simulink model "cosmic_ray_system"  (R2019a)
settings: Solver=VariableStepAuto  StartTime=0.0  StopTime=1000  RelTol=1e-3
libraries: xbsIndex_r4 x6191, casper_library_misc x163, xps_library x4, casper_library_delays x4
(part 15 of 40)

== system cosmic_ray_system/cosmic_ray/coincidence_trigger/trigger_coincidencer ==
  window_length : Inport
  data_bus_in : Inport  Port=2
  sync_in : Inport  Port=3
  adder_tree : Subsystem  AncestorBlock=casper_library_misc/adder_tree  mask(adder_tree){n_inputs=64, csp_latency=1, adder_imp=Fabric, first_stage_hdl=on, floating_point=off, dvalid_en=off, float_type=single, frac_width=0, exp_width=0}
      mask prompts: n_inputs "Number of Inputs"; csp_latency "Add Latency"; adder_imp "Adder implementation"; first_stage_hdl "Use behavioural HDL for first stage of adders"; floating_point "floating point"; float_type "float type"; frac_width "fraction length"; exp_width "exponent length"
      mask help:
      | Sums all inputs using a tree of adds and delays.
      |
      | Number of inputs: The number of inputs to the block to be summed
      | Add latency: The number of clock cycles to perform one addition (affects timing)..
      | Adder implementation: choice of fabric or DSP48E core, or behavioral HDL
      | Use behavioural HDL for first stage of adders: Causes the first stage of adders to be absorbed into DSP blocks if multipliers precede them (Virtex 5). Overrides Adder implementation
      mask init:
      | adder_tree_init(gcb, ...
      |     'n_inputs', n_inputs, ...
      |     'csp_latency', csp_latency, ...
      |     'adder_imp', adder_imp, ...
      |     'dvalid_en', dvalid_en, ...
      |     'floating_point', floating_point, ...
      |     'float_type', float_type, ...
      |     'exp_width', exp_width, ...
      |     'frac_width', frac_width, ...     
      |     'first_stage_hdl', first_stage_hdl);
      settings: AttributesFormatString=latency 6
      mask Help: eval('xlWeb(''http://casper.berkeley.edu/wiki/Adder_tree'')')
      mask TypeOptions adder_imp: Behavioral | Fabric | DSP48
      mask Callback floating_point:
      | onoff = get_param(gcb, 'floating_point');
      | if strcmp(onoff,'on')
      |     enable_fixpt = 'off'
      |     set_param_state(gcb, 'float_type', 'on')
      | 
      |     f_type = get_param(gcb, 'float_type')
      |     if strcmp(f_type,'custom')
      |         set_param_state(gcb, 'exp_width', 'on')
      |         set_param_state(gcb, 'frac_width', 'on')
      |     else
      |         set_param_state(gcb, 'exp_width', 'off')
      |         set_param_state(gcb, 'frac_width', 'off')
      |     end
      | 
      | 
      | else
      |     enable_fixpt = 'on'
      |     set_param_state(gcb, 'float_type', 'off')
      |     set_param_state(gcb, 'exp_width', 'off')
      |     set_param_state(gcb, 'frac_width', 'off')
      | end
      mask TypeOptions float_type: single | custom
      mask Callback float_type:
      | f_type = get_param(gcb, 'float_type')
      | if strcmp(f_type,'custom')
      |     set_param_state(gcb, 'exp_width', 'on')
      |     set_param_state(gcb, 'frac_width', 'on')
      | else
      |     set_param_state(gcb, 'exp_width', 'off')
      |     set_param_state(gcb, 'frac_width', 'off')
      | end
  bus_expand : Subsystem  AncestorBlock=casper_library_flow_control/bus_expand  mask(bus_expand){mode=divisions of equal size, outputNum=64, outputWidth=1, outputBinaryPt=0, outputArithmeticType=0, show_format=off, outputToWorkspace=off, variablePrefix=out, outputToModelAsWell=on}
      mask prompts: outputNum "Number of outputs:"; outputWidth "Output width:"; outputBinaryPt "Output binary point position:"; outputArithmeticType "Output arithmetic type (ufix=0, fix=1, bool=2):"; show_format "Print format string?"; outputToWorkspace "Output to workspace?"; variablePrefix "Variable name prefix:"; outputToModelAsWell "Output to model as well?"
      mask help:
      | Expands a 'bus' made using a bus_create or Xilinx
      | concat block.
      | The input will be divided into the specified number
      | of outputs with the specified arithmetic types.
      | Divisions are made from most significant bit.
      mask init: same as cosmic_ray_system/cosmic_ray/buffer_and_packetizer/bus_expand1
      settings: AttributesFormatString=64 outputs
      mask TypeOptions mode: divisions of equal size | divisions of arbitrary size
      mask Callback mode: bus_expand_callback();
      mask Callback outputWidth: bus_expand_callback();
      mask Callback outputToWorkspace: bus_expand_callback();
  custom_pulse_extend1 : Subsystem
  custom_pulse_extend10 : Subsystem
  custom_pulse_extend11 : Subsystem
  custom_pulse_extend12 : Subsystem
  custom_pulse_extend13 : Subsystem
  custom_pulse_extend14 : Subsystem
  custom_pulse_extend15 : Subsystem
  custom_pulse_extend16 : Subsystem
  custom_pulse_extend17 : Subsystem
  custom_pulse_extend18 : Subsystem
  custom_pulse_extend19 : Subsystem
  custom_pulse_extend2 : Subsystem
  custom_pulse_extend20 : Subsystem
  custom_pulse_extend21 : Subsystem
  custom_pulse_extend22 : Subsystem
  custom_pulse_extend23 : Subsystem
  custom_pulse_extend24 : Subsystem
  custom_pulse_extend25 : Subsystem
  custom_pulse_extend26 : Subsystem
  custom_pulse_extend27 : Subsystem
  custom_pulse_extend28 : Subsystem
  custom_pulse_extend29 : Subsystem
  custom_pulse_extend3 : Subsystem
  custom_pulse_extend30 : Subsystem
  custom_pulse_extend31 : Subsystem
  custom_pulse_extend32 : Subsystem
  custom_pulse_extend33 : Subsystem
  custom_pulse_extend34 : Subsystem
  custom_pulse_extend35 : Subsystem
  custom_pulse_extend36 : Subsystem
  custom_pulse_extend37 : Subsystem
  custom_pulse_extend38 : Subsystem
  custom_pulse_extend39 : Subsystem
  custom_pulse_extend4 : Subsystem
  custom_pulse_extend40 : Subsystem
  custom_pulse_extend41 : Subsystem
  custom_pulse_extend42 : Subsystem
  custom_pulse_extend43 : Subsystem
  custom_pulse_extend44 : Subsystem
  custom_pulse_extend45 : Subsystem
  custom_pulse_extend46 : Subsystem
  custom_pulse_extend47 : Subsystem
  custom_pulse_extend48 : Subsystem
  custom_pulse_extend49 : Subsystem
  custom_pulse_extend5 : Subsystem
  custom_pulse_extend50 : Subsystem
  custom_pulse_extend51 : Subsystem
  custom_pulse_extend52 : Subsystem
  custom_pulse_extend53 : Subsystem
  custom_pulse_extend54 : Subsystem
  custom_pulse_extend55 : Subsystem
  custom_pulse_extend56 : Subsystem
  custom_pulse_extend57 : Subsystem
  custom_pulse_extend58 : Subsystem
  custom_pulse_extend59 : Subsystem
  custom_pulse_extend6 : Subsystem
  custom_pulse_extend60 : Subsystem
  custom_pulse_extend61 : Subsystem
  custom_pulse_extend62 : Subsystem
  custom_pulse_extend63 : Subsystem
  custom_pulse_extend7 : Subsystem
  custom_pulse_extend8 : Subsystem
  custom_pulse_extend9 : Subsystem
  custom_pulse_extend_with_sync2 : Subsystem
  sync_out : Outport
  "out " : Outport  Port=2
  wires:
  bus_expand/24(out41) -> custom_pulse_extend20/1("in ")
  bus_expand/46(out19) -> custom_pulse_extend44/1("in ")
  custom_pulse_extend60/1("out ") -> adder_tree/62(din61)
  bus_expand/16(out49) -> custom_pulse_extend16/1("in ")
  custom_pulse_extend36/1("out ") -> adder_tree/39(din38)
  bus_expand/12(out53) -> custom_pulse_extend10/1("in ")
  bus_expand/7(out58) -> custom_pulse_extend5/1("in ")
  custom_pulse_extend32/1("out ") -> adder_tree/35(din34)
  bus_expand/23(out42) -> custom_pulse_extend23/1("in ")
  bus_expand/63(out2) -> custom_pulse_extend62/1("in ")
  bus_expand/1(msb_out64) -> custom_pulse_extend_with_sync2/1("in ")
  custom_pulse_extend6/1("out ") -> adder_tree/9(din8)
  bus_expand/2(out63) -> custom_pulse_extend46/1("in ")
  bus_expand/39(out26) -> custom_pulse_extend37/1("in ")
  custom_pulse_extend3/1("out ") -> adder_tree/6(din5)
  bus_expand/17(out48) -> custom_pulse_extend17/1("in ")
  bus_expand/42(out23) -> custom_pulse_extend40/1("in ")
  bus_expand/18(out47) -> custom_pulse_extend18/1("in ")
  bus_expand/19(out46) -> custom_pulse_extend19/1("in ")
  bus_expand/20(out45) -> custom_pulse_extend12/1("in ")
  custom_pulse_extend39/1("out ") -> adder_tree/42(din41)
  custom_pulse_extend33/1("out ") -> adder_tree/36(din35)
  custom_pulse_extend58/1("out ") -> adder_tree/60(din59)
  custom_pulse_extend8/1("out ") -> adder_tree/11(din10)
  bus_expand/49(out16) -> custom_pulse_extend48/1("in ")
  bus_expand/11(out54) -> custom_pulse_extend9/1("in ")
  custom_pulse_extend51/1("out ") -> adder_tree/53(din52)
  bus_expand/14(out51) -> custom_pulse_extend14/1("in ")
  custom_pulse_extend18/1("out ") -> adder_tree/19(din18)
  bus_expand/54(out11) -> custom_pulse_extend53/1("in ")
  bus_expand/25(out40) -> custom_pulse_extend21/1("in ")
  bus_expand/33(out32) -> custom_pulse_extend29/1("in ")
  bus_expand/53(out12) -> custom_pulse_extend52/1("in ")
  bus_expand/37(out28) -> custom_pulse_extend35/1("in ")
  bus_expand/22(out43) -> custom_pulse_extend22/1("in ")
  custom_pulse_extend31/1("out ") -> adder_tree/32(din31)
  bus_expand/51(out14) -> custom_pulse_extend50/1("in ")
  custom_pulse_extend56/1("out ") -> adder_tree/58(din57)
  custom_pulse_extend45/1("out ") -> adder_tree/48(din47)
  bus_expand/31(out34) -> custom_pulse_extend31/1("in ")
  custom_pulse_extend2/1("out ") -> adder_tree/5(din4)
  bus_expand/21(out44) -> custom_pulse_extend13/1("in ")
  bus_expand/57(out8) -> custom_pulse_extend56/1("in ")
  custom_pulse_extend22/1("out ") -> adder_tree/23(din22)
  custom_pulse_extend20/1("out ") -> adder_tree/25(din24)
  custom_pulse_extend17/1("out ") -> adder_tree/18(din17)
  custom_pulse_extend23/1("out ") -> adder_tree/24(din23)
  bus_expand/27(out38) -> custom_pulse_extend27/1("in ")
  custom_pulse_extend34/1("out ") -> adder_tree/37(din36)
  bus_expand/43(out22) -> custom_pulse_extend41/1("in ")
  custom_pulse_extend35/1("out ") -> adder_tree/38(din37)
  bus_expand/58(out7) -> custom_pulse_extend57/1("in ")
  custom_pulse_extend7/1("out ") -> adder_tree/10(din9)
  bus_expand/35(out30) -> custom_pulse_extend33/1("in ")
  bus_expand/36(out29) -> custom_pulse_extend34/1("in ")
  custom_pulse_extend21/1("out ") -> adder_tree/26(din25)
  bus_expand/60(out5) -> custom_pulse_extend59/1("in ")
  custom_pulse_extend13/1("out ") -> adder_tree/22(din21)
  bus_expand/13(out52) -> custom_pulse_extend11/1("in ")
  bus_expand/40(out25) -> custom_pulse_extend38/1("in ")
  bus_expand/52(out13) -> custom_pulse_extend51/1("in ")
  bus_expand/15(out50) -> custom_pulse_extend15/1("in ")
  custom_pulse_extend27/1("out ") -> adder_tree/28(din27)
  bus_expand/59(out6) -> custom_pulse_extend58/1("in ")
  bus_expand/29(out36) -> custom_pulse_extend25/1("in ")
  custom_pulse_extend28/1("out ") -> adder_tree/33(din32)
  window_length/1 -> custom_pulse_extend46/2("pulse_length "), custom_pulse_extend1/2("pulse_length "), custom_pulse_extend2/2("pulse_length "), custom_pulse_extend4/2("pulse_length "), custom_pulse_extend6/2("pulse_length "), custom_pulse_extend7/2("pulse_length "), custom_pulse_extend9/2("pulse_length "), custom_pulse_extend11/2("pulse_length "), custom_pulse_extend14/2("pulse_length "), custom_pulse_extend15/2("pulse_length "), custom_pulse_extend16/2("pulse_length "), custom_pulse_extend17/2("pulse_length "), custom_pulse_extend18/2("pulse_length "), custom_pulse_extend19/2("pulse_length "), custom_pulse_extend12/2("pulse_length "), custom_pulse_extend13/2("pulse_length "), custom_pulse_extend22/2("pulse_length "), custom_pulse_extend23/2("pulse_length "), custom_pulse_extend20/2("pulse_length "), custom_pulse_extend21/2("pulse_length "), custom_pulse_extend26/2("pulse_length "), custom_pulse_extend24/2("pulse_length "), custom_pulse_extend25/2("pulse_length "), custom_pulse_extend30/2("pulse_length "), custom_pulse_extend31/2("pulse_length "), custom_pulse_extend28/2("pulse_length "), custom_pulse_extend29/2("pulse_length "), custom_pulse_extend32/2("pulse_length "), custom_pulse_extend33/2("pulse_length "), custom_pulse_extend35/2("pulse_length "), custom_pulse_extend36/2("pulse_length "), custom_pulse_extend37/2("pulse_length "), custom_pulse_extend39/2("pulse_length "), custom_pulse_extend40/2("pulse_length "), custom_pulse_extend41/2("pulse_length "), custom_pulse_extend42/2("pulse_length "), custom_pulse_extend45/2("pulse_length "), custom_pulse_extend47/2("pulse_length "), custom_pulse_extend48/2("pulse_length "), custom_pulse_extend50/2("pulse_length "), custom_pulse_extend51/2("pulse_length "), custom_pulse_extend52/2("pulse_length "), custom_pulse_extend53/2("pulse_length "), custom_pulse_extend54/2("pulse_length "), custom_pulse_extend55/2("pulse_length "), custom_pulse_extend56/2("pulse_length "), custom_pulse_extend57/2("pulse_length "), custom_pulse_extend63/2("pulse_length "), custom_pulse_extend62/2("pulse_length "), custom_pulse_extend61/2("pulse_length "), custom_pulse_extend60/2("pulse_length "), custom_pulse_extend59/2("pulse_length "), custom_pulse_extend58/2("pulse_length "), custom_pulse_extend49/2("pulse_length "), custom_pulse_extend44/2("pulse_length "), custom_pulse_extend43/2("pulse_length "), custom_pulse_extend38/2("pulse_length "), custom_pulse_extend34/2("pulse_length "), custom_pulse_extend27/2("pulse_length "), custom_pulse_extend10/2("pulse_length "), custom_pulse_extend8/2("pulse_length "), custom_pulse_extend5/2("pulse_length "), custom_pulse_extend3/2("pulse_length "), custom_pulse_extend_with_sync2/2("pulse_length ")
  custom_pulse_extend_with_sync2/1("out ") -> adder_tree/2(din1)
  custom_pulse_extend4/1("out ") -> adder_tree/7(din6)
  custom_pulse_extend12/1("out ") -> adder_tree/21(din20)
  bus_expand/44(out21) -> custom_pulse_extend42/1("in ")
  custom_pulse_extend62/1("out ") -> adder_tree/64(din63)
  bus_expand/56(out9) -> custom_pulse_extend55/1("in ")
  custom_pulse_extend5/1("out ") -> adder_tree/8(din7)
  bus_expand/62(out3) -> custom_pulse_extend61/1("in ")
  bus_expand/10(out55) -> custom_pulse_extend8/1("in ")
  custom_pulse_extend19/1("out ") -> adder_tree/20(din19)
  custom_pulse_extend9/1("out ") -> adder_tree/12(din11)
  custom_pulse_extend53/1("out ") -> adder_tree/55(din54)
  data_bus_in/1 -> bus_expand/1(bus_in)
  custom_pulse_extend48/1("out ") -> adder_tree/50(din49)
  custom_pulse_extend47/1("out ") -> adder_tree/49(din48)
  bus_expand/6(out59) -> custom_pulse_extend4/1("in ")
  bus_expand/28(out37) -> custom_pulse_extend24/1("in ")
  adder_tree/2(dout) -> "out "/1
  sync_in/1 -> custom_pulse_extend_with_sync2/3(sync_in)
  custom_pulse_extend59/1("out ") -> adder_tree/61(din60)
  bus_expand/32(out33) -> custom_pulse_extend28/1("in ")
  bus_expand/47(out18) -> custom_pulse_extend45/1("in ")
  bus_expand/48(out17) -> custom_pulse_extend47/1("in ")
  custom_pulse_extend40/1("out ") -> adder_tree/43(din42)
  custom_pulse_extend57/1("out ") -> adder_tree/59(din58)
  custom_pulse_extend37/1("out ") -> adder_tree/40(din39)
  custom_pulse_extend49/1("out ") -> adder_tree/51(din50)
  bus_expand/64(lsb_out1) -> custom_pulse_extend63/1("in ")
  custom_pulse_extend25/1("out ") -> adder_tree/30(din29)
  bus_expand/34(out31) -> custom_pulse_extend32/1("in ")
  bus_expand/9(out56) -> custom_pulse_extend7/1("in ")
  custom_pulse_extend24/1("out ") -> adder_tree/29(din28)
  bus_expand/30(out35) -> custom_pulse_extend30/1("in ")
  bus_expand/5(out60) -> custom_pulse_extend3/1("in ")
  bus_expand/55(out10) -> custom_pulse_extend54/1("in ")
  custom_pulse_extend44/1("out ") -> adder_tree/47(din46)
  custom_pulse_extend11/1("out ") -> adder_tree/14(din13)
  custom_pulse_extend10/1("out ") -> adder_tree/13(din12)
  bus_expand/8(out57) -> custom_pulse_extend6/1("in ")
  custom_pulse_extend29/1("out ") -> adder_tree/34(din33)
  bus_expand/41(out24) -> custom_pulse_extend39/1("in ")
  bus_expand/61(out4) -> custom_pulse_extend60/1("in ")
  custom_pulse_extend26/1("out ") -> adder_tree/27(din26)
  bus_expand/4(out61) -> custom_pulse_extend2/1("in ")
  bus_expand/38(out27) -> custom_pulse_extend36/1("in ")
  bus_expand/45(out20) -> custom_pulse_extend43/1("in ")
  custom_pulse_extend52/1("out ") -> adder_tree/54(din53)
  custom_pulse_extend15/1("out ") -> adder_tree/16(din15)
  bus_expand/3(out62) -> custom_pulse_extend1/1("in ")
  custom_pulse_extend54/1("out ") -> adder_tree/56(din55)
  bus_expand/26(out39) -> custom_pulse_extend26/1("in ")
  adder_tree/1(sync_out) -> sync_out/1
  custom_pulse_extend30/1("out ") -> adder_tree/31(din30)
  bus_expand/50(out15) -> custom_pulse_extend49/1("in ")
  custom_pulse_extend43/1("out ") -> adder_tree/46(din45)
  custom_pulse_extend38/1("out ") -> adder_tree/41(din40)
  custom_pulse_extend16/1("out ") -> adder_tree/17(din16)
  custom_pulse_extend55/1("out ") -> adder_tree/57(din56)
  custom_pulse_extend14/1("out ") -> adder_tree/15(din14)
  custom_pulse_extend41/1("out ") -> adder_tree/44(din43)
  custom_pulse_extend42/1("out ") -> adder_tree/45(din44)
  custom_pulse_extend1/1("out ") -> adder_tree/4(din3)
  custom_pulse_extend46/1("out ") -> adder_tree/3(din2)
  custom_pulse_extend50/1("out ") -> adder_tree/52(din51)
  custom_pulse_extend61/1("out ") -> adder_tree/63(din62)
  custom_pulse_extend_with_sync2/2(sync_out) -> adder_tree/1(sync)
  custom_pulse_extend63/1("out ") -> adder_tree/65(din64)

== system cosmic_ray_system/cosmic_ray/coincidence_trigger/veto_coincidencer ==
  window_length : Inport
  data_bus_in : Inport  Port=2
  sync_in : Inport  Port=3
  adder_tree : Subsystem  AncestorBlock=casper_library_misc/adder_tree  mask(adder_tree){n_inputs=64, csp_latency=1, adder_imp=Fabric, first_stage_hdl=on, floating_point=off, dvalid_en=off, float_type=single, frac_width=0, exp_width=0}
      mask prompts: n_inputs "Number of Inputs"; csp_latency "Add Latency"; adder_imp "Adder implementation"; first_stage_hdl "Use behavioural HDL for first stage of adders"; floating_point "floating point"; float_type "float type"; frac_width "fraction length"; exp_width "exponent length"
      mask help:
      | Sums all inputs using a tree of adds and delays.
      |
      | Number of inputs: The number of inputs to the block to be summed
      | Add latency: The number of clock cycles to perform one addition (affects timing)..
      | Adder implementation: choice of fabric or DSP48E core, or behavioral HDL
      | Use behavioural HDL for first stage of adders: Causes the first stage of adders to be absorbed into DSP blocks if multipliers precede them (Virtex 5). Overrides Adder implementation
      mask init: same as cosmic_ray_system/cosmic_ray/coincidence_trigger/trigger_coincidencer/adder_tree
      settings: AttributesFormatString=latency 6
      mask Help: eval('xlWeb(''http://casper.berkeley.edu/wiki/Adder_tree'')')
      mask TypeOptions adder_imp: Behavioral | Fabric | DSP48
      mask Callback floating_point:
      | onoff = get_param(gcb, 'floating_point');
      | if strcmp(onoff,'on')
      |     enable_fixpt = 'off'
      |     set_param_state(gcb, 'float_type', 'on')
      | 
      |     f_type = get_param(gcb, 'float_type')
      |     if strcmp(f_type,'custom')
      |         set_param_state(gcb, 'exp_width', 'on')
      |         set_param_state(gcb, 'frac_width', 'on')
      |     else
      |         set_param_state(gcb, 'exp_width', 'off')
      |         set_param_state(gcb, 'frac_width', 'off')
      |     end
      | 
      | 
      | else
      |     enable_fixpt = 'on'
      |     set_param_state(gcb, 'float_type', 'off')
      |     set_param_state(gcb, 'exp_width', 'off')
      |     set_param_state(gcb, 'frac_width', 'off')
      | end
      mask TypeOptions float_type: single | custom
      mask Callback float_type:
      | f_type = get_param(gcb, 'float_type')
      | if strcmp(f_type,'custom')
      |     set_param_state(gcb, 'exp_width', 'on')
      |     set_param_state(gcb, 'frac_width', 'on')
      | else
      |     set_param_state(gcb, 'exp_width', 'off')
      |     set_param_state(gcb, 'frac_width', 'off')
      | end
  bus_expand : Subsystem  AncestorBlock=casper_library_flow_control/bus_expand  mask(bus_expand){mode=divisions of equal size, outputNum=64, outputWidth=1, outputBinaryPt=0, outputArithmeticType=0, show_format=off, outputToWorkspace=off, variablePrefix=out, outputToModelAsWell=on}
      mask prompts: outputNum "Number of outputs:"; outputWidth "Output width:"; outputBinaryPt "Output binary point position:"; outputArithmeticType "Output arithmetic type (ufix=0, fix=1, bool=2):"; show_format "Print format string?"; outputToWorkspace "Output to workspace?"; variablePrefix "Variable name prefix:"; outputToModelAsWell "Output to model as well?"
      mask help:
      | Expands a 'bus' made using a bus_create or Xilinx
      | concat block.
      | The input will be divided into the specified number
      | of outputs with the specified arithmetic types.
      | Divisions are made from most significant bit.
      mask init: same as cosmic_ray_system/cosmic_ray/buffer_and_packetizer/bus_expand1
      settings: AttributesFormatString=64 outputs
      mask TypeOptions mode: divisions of equal size | divisions of arbitrary size
      mask Callback mode: bus_expand_callback();
      mask Callback outputWidth: bus_expand_callback();
      mask Callback outputToWorkspace: bus_expand_callback();
  custom_pulse_extend1 : Subsystem
  custom_pulse_extend10 : Subsystem
  custom_pulse_extend11 : Subsystem
  custom_pulse_extend12 : Subsystem
  custom_pulse_extend13 : Subsystem
  custom_pulse_extend14 : Subsystem
  custom_pulse_extend15 : Subsystem
  custom_pulse_extend16 : Subsystem
  custom_pulse_extend17 : Subsystem
  custom_pulse_extend18 : Subsystem
  custom_pulse_extend19 : Subsystem
  custom_pulse_extend2 : Subsystem
  custom_pulse_extend20 : Subsystem
  custom_pulse_extend21 : Subsystem
  custom_pulse_extend22 : Subsystem
  custom_pulse_extend23 : Subsystem
  custom_pulse_extend24 : Subsystem
  custom_pulse_extend25 : Subsystem
  custom_pulse_extend26 : Subsystem
  custom_pulse_extend27 : Subsystem
  custom_pulse_extend28 : Subsystem
  custom_pulse_extend29 : Subsystem
  custom_pulse_extend3 : Subsystem
  custom_pulse_extend30 : Subsystem
  custom_pulse_extend31 : Subsystem
  custom_pulse_extend32 : Subsystem
  custom_pulse_extend33 : Subsystem
  custom_pulse_extend34 : Subsystem
  custom_pulse_extend35 : Subsystem
  custom_pulse_extend36 : Subsystem
  custom_pulse_extend37 : Subsystem
  custom_pulse_extend38 : Subsystem
  custom_pulse_extend39 : Subsystem
  custom_pulse_extend4 : Subsystem
  custom_pulse_extend40 : Subsystem
  custom_pulse_extend41 : Subsystem
  custom_pulse_extend42 : Subsystem
  custom_pulse_extend43 : Subsystem
  custom_pulse_extend44 : Subsystem
  custom_pulse_extend45 : Subsystem
  custom_pulse_extend46 : Subsystem
  custom_pulse_extend47 : Subsystem
  custom_pulse_extend48 : Subsystem
  custom_pulse_extend49 : Subsystem
  custom_pulse_extend5 : Subsystem
  custom_pulse_extend50 : Subsystem
  custom_pulse_extend51 : Subsystem
  custom_pulse_extend52 : Subsystem
  custom_pulse_extend53 : Subsystem
  custom_pulse_extend54 : Subsystem
  custom_pulse_extend55 : Subsystem
  custom_pulse_extend56 : Subsystem
  custom_pulse_extend57 : Subsystem
  custom_pulse_extend58 : Subsystem
  custom_pulse_extend59 : Subsystem
  custom_pulse_extend6 : Subsystem
  custom_pulse_extend60 : Subsystem
  custom_pulse_extend61 : Subsystem
  custom_pulse_extend62 : Subsystem
  custom_pulse_extend63 : Subsystem
  custom_pulse_extend7 : Subsystem
  custom_pulse_extend8 : Subsystem
  custom_pulse_extend9 : Subsystem
  custom_pulse_extend_with_sync2 : Subsystem
  sync_out : Outport
  "out " : Outport  Port=2
  wires:
  custom_pulse_extend63/1("out ") -> adder_tree/65(din64)
  custom_pulse_extend_with_sync2/2(sync_out) -> adder_tree/1(sync)
  custom_pulse_extend61/1("out ") -> adder_tree/63(din62)
  custom_pulse_extend50/1("out ") -> adder_tree/52(din51)
  custom_pulse_extend46/1("out ") -> adder_tree/3(din2)
  custom_pulse_extend1/1("out ") -> adder_tree/4(din3)
  custom_pulse_extend42/1("out ") -> adder_tree/45(din44)
  custom_pulse_extend41/1("out ") -> adder_tree/44(din43)
  custom_pulse_extend14/1("out ") -> adder_tree/15(din14)
  custom_pulse_extend55/1("out ") -> adder_tree/57(din56)
  custom_pulse_extend16/1("out ") -> adder_tree/17(din16)
  custom_pulse_extend38/1("out ") -> adder_tree/41(din40)
  custom_pulse_extend43/1("out ") -> adder_tree/46(din45)
  bus_expand/50(out15) -> custom_pulse_extend49/1("in ")
  custom_pulse_extend30/1("out ") -> adder_tree/31(din30)
  adder_tree/1(sync_out) -> sync_out/1
  bus_expand/26(out39) -> custom_pulse_extend26/1("in ")
  custom_pulse_extend54/1("out ") -> adder_tree/56(din55)
  bus_expand/3(out62) -> custom_pulse_extend1/1("in ")
  custom_pulse_extend15/1("out ") -> adder_tree/16(din15)
  custom_pulse_extend52/1("out ") -> adder_tree/54(din53)
  bus_expand/45(out20) -> custom_pulse_extend43/1("in ")
  bus_expand/38(out27) -> custom_pulse_extend36/1("in ")
  bus_expand/4(out61) -> custom_pulse_extend2/1("in ")
  custom_pulse_extend26/1("out ") -> adder_tree/27(din26)
  bus_expand/61(out4) -> custom_pulse_extend60/1("in ")
  bus_expand/41(out24) -> custom_pulse_extend39/1("in ")
  custom_pulse_extend29/1("out ") -> adder_tree/34(din33)
  bus_expand/8(out57) -> custom_pulse_extend6/1("in ")
  custom_pulse_extend10/1("out ") -> adder_tree/13(din12)
  custom_pulse_extend11/1("out ") -> adder_tree/14(din13)
  custom_pulse_extend44/1("out ") -> adder_tree/47(din46)
  bus_expand/55(out10) -> custom_pulse_extend54/1("in ")
  bus_expand/5(out60) -> custom_pulse_extend3/1("in ")
  bus_expand/30(out35) -> custom_pulse_extend30/1("in ")
  custom_pulse_extend24/1("out ") -> adder_tree/29(din28)
  bus_expand/9(out56) -> custom_pulse_extend7/1("in ")
  bus_expand/34(out31) -> custom_pulse_extend32/1("in ")
  custom_pulse_extend25/1("out ") -> adder_tree/30(din29)
  bus_expand/64(lsb_out1) -> custom_pulse_extend63/1("in ")
  custom_pulse_extend49/1("out ") -> adder_tree/51(din50)
  custom_pulse_extend37/1("out ") -> adder_tree/40(din39)
  custom_pulse_extend57/1("out ") -> adder_tree/59(din58)
  custom_pulse_extend40/1("out ") -> adder_tree/43(din42)
  bus_expand/48(out17) -> custom_pulse_extend47/1("in ")
  bus_expand/47(out18) -> custom_pulse_extend45/1("in ")
  bus_expand/32(out33) -> custom_pulse_extend28/1("in ")
  custom_pulse_extend59/1("out ") -> adder_tree/61(din60)
  sync_in/1 -> custom_pulse_extend_with_sync2/3(sync_in)
  adder_tree/2(dout) -> "out "/1
  bus_expand/28(out37) -> custom_pulse_extend24/1("in ")
  bus_expand/6(out59) -> custom_pulse_extend4/1("in ")
  custom_pulse_extend47/1("out ") -> adder_tree/49(din48)
  custom_pulse_extend48/1("out ") -> adder_tree/50(din49)
  data_bus_in/1 -> bus_expand/1(bus_in)
  custom_pulse_extend53/1("out ") -> adder_tree/55(din54)
  custom_pulse_extend9/1("out ") -> adder_tree/12(din11)
  custom_pulse_extend19/1("out ") -> adder_tree/20(din19)
  bus_expand/10(out55) -> custom_pulse_extend8/1("in ")
  bus_expand/62(out3) -> custom_pulse_extend61/1("in ")
  custom_pulse_extend5/1("out ") -> adder_tree/8(din7)
  bus_expand/56(out9) -> custom_pulse_extend55/1("in ")
  custom_pulse_extend62/1("out ") -> adder_tree/64(din63)
  bus_expand/44(out21) -> custom_pulse_extend42/1("in ")
  custom_pulse_extend12/1("out ") -> adder_tree/21(din20)
  custom_pulse_extend4/1("out ") -> adder_tree/7(din6)
  custom_pulse_extend_with_sync2/1("out ") -> adder_tree/2(din1)
  window_length/1 -> custom_pulse_extend_with_sync2/2("pulse_length "), custom_pulse_extend3/2("pulse_length "), custom_pulse_extend5/2("pulse_length "), custom_pulse_extend8/2("pulse_length "), custom_pulse_extend10/2("pulse_length "), custom_pulse_extend27/2("pulse_length "), custom_pulse_extend34/2("pulse_length "), custom_pulse_extend38/2("pulse_length "), custom_pulse_extend43/2("pulse_length "), custom_pulse_extend44/2("pulse_length "), custom_pulse_extend49/2("pulse_length "), custom_pulse_extend58/2("pulse_length "), custom_pulse_extend59/2("pulse_length "), custom_pulse_extend60/2("pulse_length "), custom_pulse_extend61/2("pulse_length "), custom_pulse_extend62/2("pulse_length "), custom_pulse_extend63/2("pulse_length "), custom_pulse_extend57/2("pulse_length "), custom_pulse_extend56/2("pulse_length "), custom_pulse_extend55/2("pulse_length "), custom_pulse_extend54/2("pulse_length "), custom_pulse_extend53/2("pulse_length "), custom_pulse_extend52/2("pulse_length "), custom_pulse_extend51/2("pulse_length "), custom_pulse_extend50/2("pulse_length "), custom_pulse_extend48/2("pulse_length "), custom_pulse_extend47/2("pulse_length "), custom_pulse_extend45/2("pulse_length "), custom_pulse_extend42/2("pulse_length "), custom_pulse_extend41/2("pulse_length "), custom_pulse_extend40/2("pulse_length "), custom_pulse_extend39/2("pulse_length "), custom_pulse_extend37/2("pulse_length "), custom_pulse_extend36/2("pulse_length "), custom_pulse_extend35/2("pulse_length "), custom_pulse_extend33/2("pulse_length "), custom_pulse_extend32/2("pulse_length "), custom_pulse_extend29/2("pulse_length "), custom_pulse_extend28/2("pulse_length "), custom_pulse_extend31/2("pulse_length "), custom_pulse_extend30/2("pulse_length "), custom_pulse_extend25/2("pulse_length "), custom_pulse_extend24/2("pulse_length "), custom_pulse_extend26/2("pulse_length "), custom_pulse_extend21/2("pulse_length "), custom_pulse_extend20/2("pulse_length "), custom_pulse_extend23/2("pulse_length "), custom_pulse_extend22/2("pulse_length "), custom_pulse_extend13/2("pulse_length "), custom_pulse_extend12/2("pulse_length "), custom_pulse_extend19/2("pulse_length "), custom_pulse_extend18/2("pulse_length "), custom_pulse_extend17/2("pulse_length "), custom_pulse_extend16/2("pulse_length "), custom_pulse_extend15/2("pulse_length "), custom_pulse_extend14/2("pulse_length "), custom_pulse_extend11/2("pulse_length "), custom_pulse_extend9/2("pulse_length "), custom_pulse_extend7/2("pulse_length "), custom_pulse_extend6/2("pulse_length "), custom_pulse_extend4/2("pulse_length "), custom_pulse_extend2/2("pulse_length "), custom_pulse_extend1/2("pulse_length "), custom_pulse_extend46/2("pulse_length ")
  custom_pulse_extend28/1("out ") -> adder_tree/33(din32)
  bus_expand/29(out36) -> custom_pulse_extend25/1("in ")
  bus_expand/59(out6) -> custom_pulse_extend58/1("in ")
  custom_pulse_extend27/1("out ") -> adder_tree/28(din27)
  bus_expand/15(out50) -> custom_pulse_extend15/1("in ")
  bus_expand/52(out13) -> custom_pulse_extend51/1("in ")
  bus_expand/40(out25) -> custom_pulse_extend38/1("in ")
  bus_expand/13(out52) -> custom_pulse_extend11/1("in ")
  custom_pulse_extend13/1("out ") -> adder_tree/22(din21)
  bus_expand/60(out5) -> custom_pulse_extend59/1("in ")
  custom_pulse_extend21/1("out ") -> adder_tree/26(din25)
  bus_expand/36(out29) -> custom_pulse_extend34/1("in ")
  bus_expand/35(out30) -> custom_pulse_extend33/1("in ")
  custom_pulse_extend7/1("out ") -> adder_tree/10(din9)
  bus_expand/58(out7) -> custom_pulse_extend57/1("in ")
  custom_pulse_extend35/1("out ") -> adder_tree/38(din37)
  bus_expand/43(out22) -> custom_pulse_extend41/1("in ")
  custom_pulse_extend34/1("out ") -> adder_tree/37(din36)
  bus_expand/27(out38) -> custom_pulse_extend27/1("in ")
  custom_pulse_extend23/1("out ") -> adder_tree/24(din23)
  custom_pulse_extend17/1("out ") -> adder_tree/18(din17)
  custom_pulse_extend20/1("out ") -> adder_tree/25(din24)
  custom_pulse_extend22/1("out ") -> adder_tree/23(din22)
  bus_expand/57(out8) -> custom_pulse_extend56/1("in ")
  bus_expand/21(out44) -> custom_pulse_extend13/1("in ")
  custom_pulse_extend2/1("out ") -> adder_tree/5(din4)
  bus_expand/31(out34) -> custom_pulse_extend31/1("in ")
  custom_pulse_extend45/1("out ") -> adder_tree/48(din47)
  custom_pulse_extend56/1("out ") -> adder_tree/58(din57)
  bus_expand/51(out14) -> custom_pulse_extend50/1("in ")
  custom_pulse_extend31/1("out ") -> adder_tree/32(din31)
  bus_expand/22(out43) -> custom_pulse_extend22/1("in ")
  bus_expand/37(out28) -> custom_pulse_extend35/1("in ")
  bus_expand/53(out12) -> custom_pulse_extend52/1("in ")
  bus_expand/33(out32) -> custom_pulse_extend29/1("in ")
  bus_expand/25(out40) -> custom_pulse_extend21/1("in ")
  bus_expand/54(out11) -> custom_pulse_extend53/1("in ")
  custom_pulse_extend18/1("out ") -> adder_tree/19(din18)
  bus_expand/14(out51) -> custom_pulse_extend14/1("in ")
  custom_pulse_extend51/1("out ") -> adder_tree/53(din52)
  bus_expand/11(out54) -> custom_pulse_extend9/1("in ")
  bus_expand/49(out16) -> custom_pulse_extend48/1("in ")
  custom_pulse_extend8/1("out ") -> adder_tree/11(din10)
  custom_pulse_extend58/1("out ") -> adder_tree/60(din59)
  custom_pulse_extend33/1("out ") -> adder_tree/36(din35)
  custom_pulse_extend39/1("out ") -> adder_tree/42(din41)
  bus_expand/20(out45) -> custom_pulse_extend12/1("in ")
  bus_expand/19(out46) -> custom_pulse_extend19/1("in ")
  bus_expand/18(out47) -> custom_pulse_extend18/1("in ")
  bus_expand/42(out23) -> custom_pulse_extend40/1("in ")
  bus_expand/17(out48) -> custom_pulse_extend17/1("in ")
  custom_pulse_extend3/1("out ") -> adder_tree/6(din5)
  bus_expand/39(out26) -> custom_pulse_extend37/1("in ")
  bus_expand/2(out63) -> custom_pulse_extend46/1("in ")
  custom_pulse_extend6/1("out ") -> adder_tree/9(din8)
  bus_expand/1(msb_out64) -> custom_pulse_extend_with_sync2/1("in ")
  bus_expand/63(out2) -> custom_pulse_extend62/1("in ")
  bus_expand/23(out42) -> custom_pulse_extend23/1("in ")
  custom_pulse_extend32/1("out ") -> adder_tree/35(din34)
  bus_expand/7(out58) -> custom_pulse_extend5/1("in ")
  bus_expand/12(out53) -> custom_pulse_extend10/1("in ")
  custom_pulse_extend36/1("out ") -> adder_tree/39(din38)
  bus_expand/16(out49) -> custom_pulse_extend16/1("in ")
  custom_pulse_extend60/1("out ") -> adder_tree/62(din61)
  bus_expand/46(out19) -> custom_pulse_extend44/1("in ")
  bus_expand/24(out41) -> custom_pulse_extend20/1("in ")

== system cosmic_ray_system/cosmic_ray/constant/bus_create1 ==
  in1 : Inport
  in2 : Inport  Port=2
  in3 : Inport  Port=3
  in4 : Inport  Port=4
  in5 : Inport  Port=5
  in6 : Inport  Port=6
  in7 : Inport  Port=7
  in8 : Inport  Port=8
  in9 : Inport  Port=9
  in10 : Inport  Port=10
  in11 : Inport  Port=11
  in12 : Inport  Port=12
  in13 : Inport  Port=13
  in14 : Inport  Port=14
  in15 : Inport  Port=15
  in16 : Inport  Port=16
  in17 : Inport  Port=17
  in18 : Inport  Port=18
  in19 : Inport  Port=19
  in20 : Inport  Port=20
  in21 : Inport  Port=21
  in22 : Inport  Port=22
  in23 : Inport  Port=23
  in24 : Inport  Port=24
  in25 : Inport  Port=25
  in26 : Inport  Port=26
  in27 : Inport  Port=27
  in28 : Inport  Port=28
  in29 : Inport  Port=29
  in30 : Inport  Port=30
  in31 : Inport  Port=31
  in32 : Inport  Port=32
  in33 : Inport  Port=33
  in34 : Inport  Port=34
  in35 : Inport  Port=35
  in36 : Inport  Port=36
  in37 : Inport  Port=37
  in38 : Inport  Port=38
  in39 : Inport  Port=39
  in40 : Inport  Port=40
  in41 : Inport  Port=41
  in42 : Inport  Port=42
  in43 : Inport  Port=43
  in44 : Inport  Port=44
  in45 : Inport  Port=45
  in46 : Inport  Port=46
  in47 : Inport  Port=47
  in48 : Inport  Port=48
  in49 : Inport  Port=49
  in50 : Inport  Port=50
  in51 : Inport  Port=51
  in52 : Inport  Port=52
  in53 : Inport  Port=53
  in54 : Inport  Port=54
  in55 : Inport  Port=55
  in56 : Inport  Port=56
  in57 : Inport  Port=57
  in58 : Inport  Port=58
  in59 : Inport  Port=59
  in60 : Inport  Port=60
  in61 : Inport  Port=61
  in62 : Inport  Port=62
  in63 : Inport  Port=63
  in64 : Inport  Port=64
  concatenate : xbsIndex_r4/Concat  num_inputs=64  dbl_ovrd=off  block_type=concat
  reinterpret{1..64} (64 alike) : xbsIndex_r4/Reinterpret  force_arith_type=on  arith_type=Unsigned  force_bin_pt=on  bin_pt=0  block_type=reinterpret
      reinterpret1 settings: infoedit="Changes signal type without altering the binary representation.   You can changed the signal between signed and unsigned, and relocate the binary point.<br><br>Hardware notes: In hardware this block costs nothing.<br><br>Example:  Suppose the input is 6 bits wide, signed, with 2 fractional bits, and the output is forced to unsigned with 0 fractional bits.  Then an input of -2.0 (1110.00 in binary 2's complement) becomes an output of 56 (111000 in binary)."
      reinterpret2 settings: infoedit="Changes signal type without altering the binary representation.   You can changed the signal between signed and unsigned, and relocate the binary point.<br><br>Hardware notes: In hardware this block costs nothing.<br><br>Example:  Suppose the input is 6 bits wide, signed, with 2 fractional bits, and the output is forced to unsigned with 0 fractional bits.  Then an input of -2.0 (1110.00 in binary 2's complement) becomes an output of 56 (111000 in binary)."
  bus_out : Outport
  wires:
  concatenate/1 -> bus_out/1
  in1/1 -> reinterpret1/1
  reinterpret1/1 -> concatenate/1
  in2/1 -> reinterpret2/1
  reinterpret2/1 -> concatenate/2
  in3/1 -> reinterpret3/1
  reinterpret3/1 -> concatenate/3
  in4/1 -> reinterpret4/1
  reinterpret4/1 -> concatenate/4
  in5/1 -> reinterpret5/1
  reinterpret5/1 -> concatenate/5
  in6/1 -> reinterpret6/1
  reinterpret6/1 -> concatenate/6
  in7/1 -> reinterpret7/1
  reinterpret7/1 -> concatenate/7
  in8/1 -> reinterpret8/1
  reinterpret8/1 -> concatenate/8
  in9/1 -> reinterpret9/1
  reinterpret9/1 -> concatenate/9
  in10/1 -> reinterpret10/1
  reinterpret10/1 -> concatenate/10
  in11/1 -> reinterpret11/1
  reinterpret11/1 -> concatenate/11
  in12/1 -> reinterpret12/1
  reinterpret12/1 -> concatenate/12
  in13/1 -> reinterpret13/1
  reinterpret13/1 -> concatenate/13
  in14/1 -> reinterpret14/1
  reinterpret14/1 -> concatenate/14
  in15/1 -> reinterpret15/1
  reinterpret15/1 -> concatenate/15
  in16/1 -> reinterpret16/1
  reinterpret16/1 -> concatenate/16
  in17/1 -> reinterpret17/1
  reinterpret17/1 -> concatenate/17
  in18/1 -> reinterpret18/1
  reinterpret18/1 -> concatenate/18
  in19/1 -> reinterpret19/1
  reinterpret19/1 -> concatenate/19
  in20/1 -> reinterpret20/1
  reinterpret20/1 -> concatenate/20
  in21/1 -> reinterpret21/1
  reinterpret21/1 -> concatenate/21
  in22/1 -> reinterpret22/1
  reinterpret22/1 -> concatenate/22
  in23/1 -> reinterpret23/1
  reinterpret23/1 -> concatenate/23
  in24/1 -> reinterpret24/1
  reinterpret24/1 -> concatenate/24
  in25/1 -> reinterpret25/1
  reinterpret25/1 -> concatenate/25
  in26/1 -> reinterpret26/1
  reinterpret26/1 -> concatenate/26
  in27/1 -> reinterpret27/1
  reinterpret27/1 -> concatenate/27
  in28/1 -> reinterpret28/1
  reinterpret28/1 -> concatenate/28
  in29/1 -> reinterpret29/1
  reinterpret29/1 -> concatenate/29
  in30/1 -> reinterpret30/1
  reinterpret30/1 -> concatenate/30
  in31/1 -> reinterpret31/1
  reinterpret31/1 -> concatenate/31
  in32/1 -> reinterpret32/1
  reinterpret32/1 -> concatenate/32
  in33/1 -> reinterpret33/1
  reinterpret33/1 -> concatenate/33
  in34/1 -> reinterpret34/1
  reinterpret34/1 -> concatenate/34
  in35/1 -> reinterpret35/1
  reinterpret35/1 -> concatenate/35
  in36/1 -> reinterpret36/1
  reinterpret36/1 -> concatenate/36
  in37/1 -> reinterpret37/1
  reinterpret37/1 -> concatenate/37
  in38/1 -> reinterpret38/1
  reinterpret38/1 -> concatenate/38
  in39/1 -> reinterpret39/1
  reinterpret39/1 -> concatenate/39
  in40/1 -> reinterpret40/1
  reinterpret40/1 -> concatenate/40
  in41/1 -> reinterpret41/1
  reinterpret41/1 -> concatenate/41
  in42/1 -> reinterpret42/1
  reinterpret42/1 -> concatenate/42
  in43/1 -> reinterpret43/1
  reinterpret43/1 -> concatenate/43
  in44/1 -> reinterpret44/1
  reinterpret44/1 -> concatenate/44
  in45/1 -> reinterpret45/1
  reinterpret45/1 -> concatenate/45
  in46/1 -> reinterpret46/1
  reinterpret46/1 -> concatenate/46
  in47/1 -> reinterpret47/1
  reinterpret47/1 -> concatenate/47
  in48/1 -> reinterpret48/1
  reinterpret48/1 -> concatenate/48
  in49/1 -> reinterpret49/1
  reinterpret49/1 -> concatenate/49
  in50/1 -> reinterpret50/1
  reinterpret50/1 -> concatenate/50
  in51/1 -> reinterpret51/1
  reinterpret51/1 -> concatenate/51
  in52/1 -> reinterpret52/1
  reinterpret52/1 -> concatenate/52
  in53/1 -> reinterpret53/1
  reinterpret53/1 -> concatenate/53
  in54/1 -> reinterpret54/1
  reinterpret54/1 -> concatenate/54
  in55/1 -> reinterpret55/1
  reinterpret55/1 -> concatenate/55
  in56/1 -> reinterpret56/1
  reinterpret56/1 -> concatenate/56
  in57/1 -> reinterpret57/1
  reinterpret57/1 -> concatenate/57
  in58/1 -> reinterpret58/1
  reinterpret58/1 -> concatenate/58
  in59/1 -> reinterpret59/1
  reinterpret59/1 -> concatenate/59
  in60/1 -> reinterpret60/1
  reinterpret60/1 -> concatenate/60
  in61/1 -> reinterpret61/1
  reinterpret61/1 -> concatenate/61
  in62/1 -> reinterpret62/1
  reinterpret62/1 -> concatenate/62
  in63/1 -> reinterpret63/1
  reinterpret63/1 -> concatenate/63
  in64/1 -> reinterpret64/1
  reinterpret64/1 -> concatenate/64

== system cosmic_ray_system/cosmic_ray/constant_test_signal1/bus_create ==
  in1 : Inport
  in2 : Inport  Port=2
  in3 : Inport  Port=3
  in4 : Inport  Port=4
  in5 : Inport  Port=5
  in6 : Inport  Port=6
  in7 : Inport  Port=7
  in8 : Inport  Port=8
  in9 : Inport  Port=9
  in10 : Inport  Port=10
  in11 : Inport  Port=11
  in12 : Inport  Port=12
  in13 : Inport  Port=13
  in14 : Inport  Port=14
  in15 : Inport  Port=15
  in16 : Inport  Port=16
  in17 : Inport  Port=17
  in18 : Inport  Port=18
  in19 : Inport  Port=19
  in20 : Inport  Port=20
  in21 : Inport  Port=21
  in22 : Inport  Port=22
  in23 : Inport  Port=23
  in24 : Inport  Port=24
  in25 : Inport  Port=25
  in26 : Inport  Port=26
  in27 : Inport  Port=27
  in28 : Inport  Port=28
  in29 : Inport  Port=29
  in30 : Inport  Port=30
  in31 : Inport  Port=31
  in32 : Inport  Port=32
  in33 : Inport  Port=33
  in34 : Inport  Port=34
  in35 : Inport  Port=35
  in36 : Inport  Port=36
  in37 : Inport  Port=37
  in38 : Inport  Port=38
  in39 : Inport  Port=39
  in40 : Inport  Port=40
  in41 : Inport  Port=41
  in42 : Inport  Port=42
  in43 : Inport  Port=43
  in44 : Inport  Port=44
  in45 : Inport  Port=45
  in46 : Inport  Port=46
  in47 : Inport  Port=47
  in48 : Inport  Port=48
  in49 : Inport  Port=49
  in50 : Inport  Port=50
  in51 : Inport  Port=51
  in52 : Inport  Port=52
  in53 : Inport  Port=53
  in54 : Inport  Port=54
  in55 : Inport  Port=55
  in56 : Inport  Port=56
  in57 : Inport  Port=57
  in58 : Inport  Port=58
  in59 : Inport  Port=59
  in60 : Inport  Port=60
  in61 : Inport  Port=61
  in62 : Inport  Port=62
  in63 : Inport  Port=63
  in64 : Inport  Port=64
  concatenate : xbsIndex_r4/Concat  num_inputs=64  dbl_ovrd=off  block_type=concat
  reinterpret{1..64} (64 alike) : xbsIndex_r4/Reinterpret  force_arith_type=on  arith_type=Unsigned  force_bin_pt=on  bin_pt=0  block_type=reinterpret
      reinterpret1 settings: infoedit="Changes signal type without altering the binary representation.   You can changed the signal between signed and unsigned, and relocate the binary point.<br><br>Hardware notes: In hardware this block costs nothing.<br><br>Example:  Suppose the input is 6 bits wide, signed, with 2 fractional bits, and the output is forced to unsigned with 0 fractional bits.  Then an input of -2.0 (1110.00 in binary 2's complement) becomes an output of 56 (111000 in binary)."
      reinterpret2 settings: infoedit="Changes signal type without altering the binary representation.   You can changed the signal between signed and unsigned, and relocate the binary point.<br><br>Hardware notes: In hardware this block costs nothing.<br><br>Example:  Suppose the input is 6 bits wide, signed, with 2 fractional bits, and the output is forced to unsigned with 0 fractional bits.  Then an input of -2.0 (1110.00 in binary 2's complement) becomes an output of 56 (111000 in binary)."
  bus_out : Outport
  wires:
  concatenate/1 -> bus_out/1
  in1/1 -> reinterpret1/1
  reinterpret1/1 -> concatenate/1
  in2/1 -> reinterpret2/1
  reinterpret2/1 -> concatenate/2
  in3/1 -> reinterpret3/1
  reinterpret3/1 -> concatenate/3
  in4/1 -> reinterpret4/1
  reinterpret4/1 -> concatenate/4
  in5/1 -> reinterpret5/1
  reinterpret5/1 -> concatenate/5
  in6/1 -> reinterpret6/1
  reinterpret6/1 -> concatenate/6
  in7/1 -> reinterpret7/1
  reinterpret7/1 -> concatenate/7
  in8/1 -> reinterpret8/1
  reinterpret8/1 -> concatenate/8
  in9/1 -> reinterpret9/1
  reinterpret9/1 -> concatenate/9
  in10/1 -> reinterpret10/1
  reinterpret10/1 -> concatenate/10
  in11/1 -> reinterpret11/1
  reinterpret11/1 -> concatenate/11
  in12/1 -> reinterpret12/1
  reinterpret12/1 -> concatenate/12
  in13/1 -> reinterpret13/1
  reinterpret13/1 -> concatenate/13
  in14/1 -> reinterpret14/1
  reinterpret14/1 -> concatenate/14
  in15/1 -> reinterpret15/1
  reinterpret15/1 -> concatenate/15
  in16/1 -> reinterpret16/1
  reinterpret16/1 -> concatenate/16
  in17/1 -> reinterpret17/1
  reinterpret17/1 -> concatenate/17
  in18/1 -> reinterpret18/1
  reinterpret18/1 -> concatenate/18
  in19/1 -> reinterpret19/1
  reinterpret19/1 -> concatenate/19
  in20/1 -> reinterpret20/1
  reinterpret20/1 -> concatenate/20
  in21/1 -> reinterpret21/1
  reinterpret21/1 -> concatenate/21
  in22/1 -> reinterpret22/1
  reinterpret22/1 -> concatenate/22
  in23/1 -> reinterpret23/1
  reinterpret23/1 -> concatenate/23
  in24/1 -> reinterpret24/1
  reinterpret24/1 -> concatenate/24
  in25/1 -> reinterpret25/1
  reinterpret25/1 -> concatenate/25
  in26/1 -> reinterpret26/1
  reinterpret26/1 -> concatenate/26
  in27/1 -> reinterpret27/1
  reinterpret27/1 -> concatenate/27
  in28/1 -> reinterpret28/1
  reinterpret28/1 -> concatenate/28
  in29/1 -> reinterpret29/1
  reinterpret29/1 -> concatenate/29
  in30/1 -> reinterpret30/1
  reinterpret30/1 -> concatenate/30
  in31/1 -> reinterpret31/1
  reinterpret31/1 -> concatenate/31
  in32/1 -> reinterpret32/1
  reinterpret32/1 -> concatenate/32
  in33/1 -> reinterpret33/1
  reinterpret33/1 -> concatenate/33
  in34/1 -> reinterpret34/1
  reinterpret34/1 -> concatenate/34
  in35/1 -> reinterpret35/1
  reinterpret35/1 -> concatenate/35
  in36/1 -> reinterpret36/1
  reinterpret36/1 -> concatenate/36
  in37/1 -> reinterpret37/1
  reinterpret37/1 -> concatenate/37
  in38/1 -> reinterpret38/1
  reinterpret38/1 -> concatenate/38
  in39/1 -> reinterpret39/1
  reinterpret39/1 -> concatenate/39
  in40/1 -> reinterpret40/1
  reinterpret40/1 -> concatenate/40
  in41/1 -> reinterpret41/1
  reinterpret41/1 -> concatenate/41
  in42/1 -> reinterpret42/1
  reinterpret42/1 -> concatenate/42
  in43/1 -> reinterpret43/1
  reinterpret43/1 -> concatenate/43
  in44/1 -> reinterpret44/1
  reinterpret44/1 -> concatenate/44
  in45/1 -> reinterpret45/1
  reinterpret45/1 -> concatenate/45
  in46/1 -> reinterpret46/1
  reinterpret46/1 -> concatenate/46
  in47/1 -> reinterpret47/1
  reinterpret47/1 -> concatenate/47
  in48/1 -> reinterpret48/1
  reinterpret48/1 -> concatenate/48
  in49/1 -> reinterpret49/1
  reinterpret49/1 -> concatenate/49
  in50/1 -> reinterpret50/1
  reinterpret50/1 -> concatenate/50
  in51/1 -> reinterpret51/1
  reinterpret51/1 -> concatenate/51
  in52/1 -> reinterpret52/1
  reinterpret52/1 -> concatenate/52
  in53/1 -> reinterpret53/1
  reinterpret53/1 -> concatenate/53
  in54/1 -> reinterpret54/1
  reinterpret54/1 -> concatenate/54
  in55/1 -> reinterpret55/1
  reinterpret55/1 -> concatenate/55
  in56/1 -> reinterpret56/1
  reinterpret56/1 -> concatenate/56
  in57/1 -> reinterpret57/1
  reinterpret57/1 -> concatenate/57
  in58/1 -> reinterpret58/1
  reinterpret58/1 -> concatenate/58
  in59/1 -> reinterpret59/1
  reinterpret59/1 -> concatenate/59
  in60/1 -> reinterpret60/1
  reinterpret60/1 -> concatenate/60
  in61/1 -> reinterpret61/1
  reinterpret61/1 -> concatenate/61
  in62/1 -> reinterpret62/1
  reinterpret62/1 -> concatenate/62
  in63/1 -> reinterpret63/1
  reinterpret63/1 -> concatenate/63
  in64/1 -> reinterpret64/1
  reinterpret64/1 -> concatenate/64
